simulink model "c230422_FCEV_SLMP_tbSOC_FPSD_EMS4H"  (R2022b)
settings: Solver=FixedStepAuto  StartTime=0.0  StopTime=DrvCycLen  FixedStep=1  RelTol=1e-3
values from neighbouring files (symbols this model uses):
  AccThrshd = 1    [Config_c221112.m]    (also in Config_c221127.m; Config_c221218.m; Config_c230117.m; Config_c230321.m)
  AlphaRampFactor = 8    [Config_c221112.m]    (also in Config_c221127.m; Config_c221218.m; Config_c230117.m; Config_c230321.m)
  Bat_ori_SOC2 = [0 0.001 0.002 0.003 0.004 0.005 0.006 0.007 0.008 0.009 0.01 0.011 ... (1001 elements, 1x1001)]    [FCEV_original_data.mat]
  Bat_ori_Uoc_chg_V = [2.4478 2.54923264342 2.6007 2.6383 2.66953057366 2.69636321708 2.7197 2.74042850391 2.75906114733 2.77619379074 2.792 2.80675907757 ... (1001 elements, 1x1001)]    [FCEV_original_data.mat]
  Bat_ori_Uoc_dis_V = [1.9998 2.03916768329 2.24724374236 2.39700902919 2.48767431602 2.5476 2.5882 2.6202 2.64771773167 2.6719 2.6933 2.71251566192 ... (1001 elements, 1x1001)]    [FCEV_original_data.mat]
  Bat_power_max_kW = 50    [FCEV_original_data.mat]
  Bat_power_min_kW = 0    [FCEV_original_data.mat]
  Bat_SOC_min = 0.3    [FCEV_original_data.mat]
  BattOnly = 0    [Config_c221218.m]    (also in Config_c230117.m = BattSocRightNow > BattSocLowerLimit; Config_c230321.m = double(BattSocRightNow > BattSocLowerLimit))
  BattPack_current = BattCell_current * 9    (= 20.7)    [Config_c230321.m]
  BattSocInit = 0.9    [Config_c221112.m]    (also in Config_c221127.m = 0.3; Config_c221218.m = 0.3; Config_c230117.m = 0.8; Config_c230321.m = 0.8)
  BattSocLowerLimit = 0.25    [Config_c221112.m]    (also in Config_c221127.m = 0.3; Config_c221218.m = 0.3; Config_c230117.m = 0.3; Config_c230321.m = 0.3)
  BattSocRightNow = BattSocRightNow - SocDrop    [Config_c221218.m]    (also in Config_c230117.m; Config_c230321.m)
  BattSocUpperLimit = 0.9    [Config_c221112.m]    (also in Config_c221127.m = 0.8; Config_c221218.m = 0.8; Config_c230117.m = 0.8; Config_c230321.m = 0.8)
  CFWF = 0.5    [Config_c221127.m]    (also in Config_c221218.m; Config_c230117.m; Config_c230321.m)
  DCAC_eff = 0.95    [FCEV_original_data.mat]
  DCDC_ori_eff = [0.95 0.96 0.97 0.976 0.98 0.978 0.973 0.962]    [FCEV_original_data.mat]
  DCDC_ori_power_kW = [0 10 20 30 40 50 60 70]    [FCEV_original_data.mat]
  DeAccThrshd = -1    [Config_c221112.m]    (also in Config_c221127.m; Config_c221218.m; Config_c230117.m; Config_c230321.m)
  DeltaFcPwrRcm_down = 0.5    [Config_c221127.m]    (also in Config_c221218.m; Config_c230117.m; Config_c230321.m)
  DeltaFcPwrRcm_up = 2    [Config_c221127.m]    (also in Config_c221218.m = 3; Config_c230117.m = 4; Config_c230321.m = 4)
  DrvCycRange = sum(DrvCycVps(:,2))    [Config_c221112.m]    (also in Config_c221127.m; Config_c221218.m; Config_c230117.m; Config_c230321.m)
  FC_ori_eff = [0.1 0.33 0.492 0.533 0.559 0.596 0.591 0.562 0.508]    [FCEV_original_data.mat]
  FC_ori_fuel_rate_gps = [0 0.0505050505051 0.0846883468835 0.117260787992 0.149075730471 0.279642058166 0.423011844332 0.593119810202 0.820209973753]    [FCEV_original_data.mat]
  FC_ori_power_kW = [0 2 5 7.5 10 20 30 40 50]    [FCEV_original_data.mat]
  FC_power_max_kW = 50    [FCEV_original_data.mat]
  FC_power_min_kW = 0    [FCEV_original_data.mat]
  FcPwrDropCall = 6    [Config_c221127.m]    (also in Config_c221218.m; Config_c230117.m; Config_c230321.m)
  HydpriceRmb = 30    [Config_c221127.m]    (also in Config_c221218.m; Config_c230117.m; Config_c230321.m)
  m = Time_sample    [Config_c22100601.m]    (also in Config_c22100701.m)
  MC_eff_brk_average = 0.810578512397    [FCEV_original_data.mat]
  MC_eff_dri_average = 0.810578512397    [FCEV_original_data.mat]
  MC_inertia = 0.06    [FCEV_original_data.mat]
  MC_ori_eff = [0.7 0.78 0.85 0.86 0.81 0.82 0.79 0.78 0.78 0.78 0.78 0.7 ... (231 elements, 11x21)]    [FCEV_original_data.mat]
  MC_ori_power_brk_req_kW = [0 -28.3912930389 -56.7825860779 -85.1738791168 -113.565172156 -141.956465195 -170.347758234 -198.739051273 -227.130344311 -255.52163735 -283.912930389 0 ... (121 elements, 11x11)]    [FCEV_original_data.mat]
  MC_ori_power_dri_req_kW = [0 0 0 0 0 0 0 0 0 0 0 0 ... (121 elements, 11x11)]    [FCEV_original_data.mat]
  MC_ori_spd_rpm = [0 1000 2000 3000 4000 5000 6000 7000 8000 9000 10000]    [FCEV_original_data.mat]
  MC_ori_trq_brk_max_Nm = [-271.1368 -271.1368 -271.1368 -237.5159 -178.1369 -142.4824 -118.7579 -101.8119 -89.0685 -79.172 -71.1734]    [FCEV_original_data.mat]
  MC_ori_trq_brk_Nm = [-271.136848522 -244.02316367 -216.909478817 -189.795793965 -162.682109113 -135.568424261 -108.454739409 -81.3410545565 -54.2273697044 -27.1136848522 0]    [FCEV_original_data.mat]
  MC_ori_trq_dri_max_Nm = [271.1368 271.1368 271.1368 237.5159 178.1369 142.4824 118.7579 101.8119 89.0685 79.172 71.1734]    [FCEV_original_data.mat]
  MC_ori_trq_dri_Nm = [0 27.1136848522 54.2273697044 81.3410545565 108.454739409 135.568424261 162.682109113 189.795793965 216.909478817 244.02316367 271.136848522]    [FCEV_original_data.mat]
  MC_ori_trq_Nm = [-271.136848522 -244.02316367 -216.909478817 -189.795793965 -162.682109113 -135.568424261 -108.454739409 -81.3410545565 -54.2273697044 -27.1136848522 0 27.1136848522 ... (21 elements, 1x21)]    [FCEV_original_data.mat]
  MC_power_max_kW = 75    [FCEV_original_data.mat]
  MC_spd_max_rpm = 10000    [FCEV_original_data.mat]
  MC_spd_min_rpm = 0    [FCEV_original_data.mat]
  MC_spd_scale = 1    [FCEV_original_data.mat]
  MC_trq_scale = 1    [FCEV_original_data.mat]
  nbl_std = (20/nbl_btm)^(1/0.57)    [Config_c230321.m]
  no_FcPwrSlowDrop = 1    [Config_c230321.m]
  Placeholder = 0    [Config_c221127.m]    (also in Config_c221218.m; Config_c230117.m; Config_c230321.m)
  PredLen = 5    [Config_c221112.m]    (also in Config_c221127.m; Config_c221218.m; Config_c230117.m; Config_c230321.m)
  Q_batt = 20.7*3600    (= 74520)    [Config_c22100701.m]    (also in Config_c230321.m = 18000)
  Road_u = 0.75    [FCEV_original_data.mat]
  sc_E = 0.5 * C_eff * V_eff^2    (= 512000)    [Config_c230321.m]
  SC_np = 1    [Config_c230321.m]
  SC_ns = 100    [Config_c230321.m]
  SC_rc = 1000    [Config_c230321.m]
  sc_soc_init = 0.5    [Config_c230321.m]
  SFun_ipt = [sc_discharge_limit;sc_charge_limit;sc_E;Sc_pwr_upper_lmt;BattSocLowerLimit;     BattSocUpperLimit;Q_batt;BattUoc;50;]    [Config_c230321.m]
  SLMP_LearningRate = 0.05    [Config_c221112.m]    (also in Config_c221127.m; Config_c221218.m; Config_c230117.m; Config_c230321.m)
  tDegTable = [zeros(1,3),linspace(0,0.13,47)]    [Config_c221127.m]    (also in Config_c221218.m; Config_c230117.m; Config_c230321.m)
  usd2rmb = 7.116    [Config_c22100601.m]    (also in Config_c22100701.m; Config_c221106.m = 6; Config_c221112.m = 6; Config_c221127.m = 6)
  Veh_air_density_kgpm2 = 1.2    [FCEV_original_data.mat]
  Veh_brk_front = [1 0.6 0.608 0.61 0.618 0.624 0.636 0.645 0.655]    [FCEV_original_data.mat]
  Veh_brk_z = [0.1 0.2 0.3 0.4 0.5 0.6 0.7 0.8 0.9]    [FCEV_original_data.mat]
  Veh_brk_z_max = 0.7    [FCEV_original_data.mat]
  Veh_brk_z_min = 0.1    [FCEV_original_data.mat]
  Veh_coeff_drag = 0.312    [FCEV_original_data.mat]
  Veh_coeff_roll = 0.00863    [FCEV_original_data.mat]
  Veh_final_drive_inertia = 0.1105    [FCEV_original_data.mat]
  Veh_final_drive_ratio = 3.47    [FCEV_original_data.mat]
  Veh_frontal_area_m2 = 2.06    [FCEV_original_data.mat]
  Veh_gravity_acc_ms2 = 9.81    [FCEV_original_data.mat]
  Veh_mass_cargo_kg = 113    [FCEV_original_data.mat]
  Veh_mass_curb_kg = 1157    [FCEV_original_data.mat]
  Veh_mech_eff = 0.9    [FCEV_original_data.mat]
  Veh_rotary_mass_conversion_factor = 1.05    [FCEV_original_data.mat]
  Veh_size_cg_height_m = 0.53    [FCEV_original_data.mat]
  Veh_wheel_inertia = 3.1039    [FCEV_original_data.mat]
  Veh_wheel_radius_m = 0.313    [FCEV_original_data.mat]
  Veh_wt_frac_front = 0.5    [FCEV_original_data.mat]
  VstdThrshd = 2    [Config_c221112.m]    (also in Config_c221127.m; Config_c221218.m; Config_c230117.m; Config_c230321.m)
undefined symbols (not defined in the file or in its folder): Bat_ori_temp, SC_iv, SC_nm, SC_SocTable
libraries: autolibshared x2
(part 2 of 7)

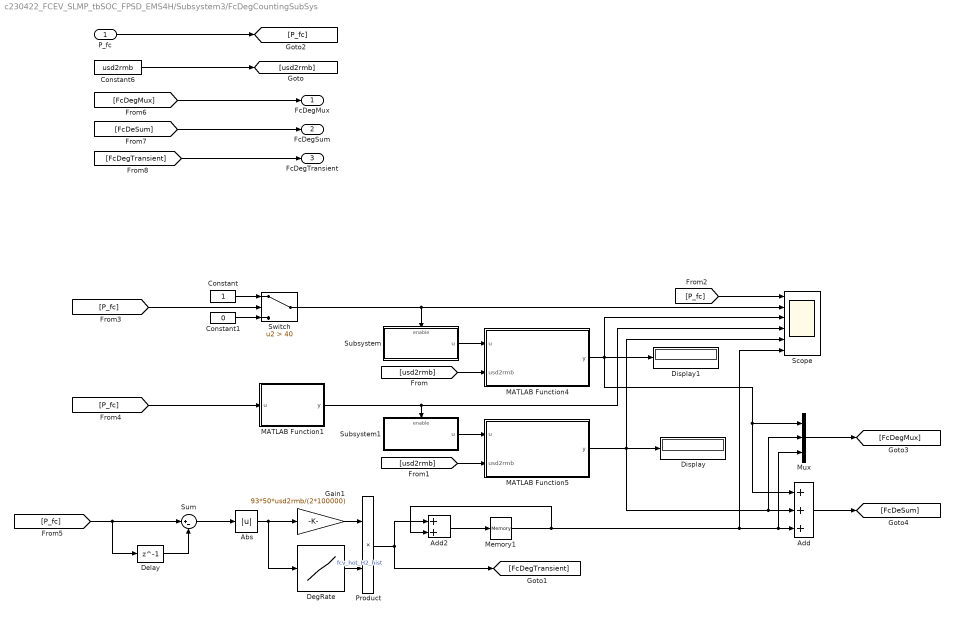
== system c230422_FCEV_SLMP_tbSOC_FPSD_EMS4H/Subsystem3/FcDegCountingSubSys ==
  P_fc : Inport
  Abs : Abs  SaturateOnIntegerOverflow=off
  Add : Sum  Inputs=+++
  Add2 : Sum
  Constant : Constant
  Constant1 : Constant  Value=0
  Constant6 : Constant  Value=usd2rmb
  DegRate : Lookup_n-D  NumberOfTableDimensions=1  BreakpointsForDimension1=1:50  Table=tDegTable  RndMeth=Simplest
  Delay : Delay  DelayLength=1
  Display : Display
  Display1 : Display
  Gain1 : Gain  Gain=93*50*usd2rmb/(2*100000)
  MATLAB Function1 : MATLAB Function  TreatAsAtomicUnit=on
  MATLAB Function4 : MATLAB Function  TreatAsAtomicUnit=on
  MATLAB Function5 : MATLAB Function  TreatAsAtomicUnit=on
  Memory1 : Memory
  Mux : Mux  Inputs=3
  Product : Product
  Scope : Scope  NumInputPorts=6
  Subsystem : Subsystem
  Subsystem1 : Subsystem
  Sum : Sum  Inputs=|+-
  Switch : Switch  Criteria=u2 > Threshold  Threshold=40  SaturateOnIntegerOverflow=off  InputSameDT=off
  FcDegMux : Outport
  FcDegSum : Outport  Port=2
  FcDegTransient : Outport  Port=3
  wires:
  MATLAB Function5/1(y) -> Scope/5, Display/1, Mux/2, Add/2
  MATLAB Function1/1(y) -> Subsystem1/Enable, Scope/4
  Subsystem/1(u) -> MATLAB Function4/1(u)
  Constant/1 -> Switch/1
  [usd2rmb] -> MATLAB Function4/2(usd2rmb)
  Constant1/1 -> Switch/3
  [usd2rmb] -> MATLAB Function5/2(usd2rmb)
  Switch/1 -> Scope/2, Subsystem/Enable
  P_fc/1 -> [P_fc]
  Subsystem1/1(u) -> MATLAB Function5/1(u)
  MATLAB Function4/1(y) -> Scope/3, Mux/1, Add/1, Display1/1
  Constant6/1 -> [usd2rmb]
  [P_fc] -> Scope/1
  Memory1/1 -> Scope/6, Mux/3, Add/3, Add2/2
  Add2/1 -> Memory1/1
  Sum/1 -> Abs/1
  Abs/1 -> DegRate/1, Gain1/1
  Delay/1 -> Sum/2
  [P_fc] -> Delay/1, Sum/1
  [P_fc] -> Switch/2
  Add/1 -> [FcDeSum]
  Mux/1 -> [FcDegMux]
  [P_fc] -> MATLAB Function1/1(u)
  [FcDegMux] -> FcDegMux/1
  [FcDeSum] -> FcDegSum/1
  [FcDegTransient] -> FcDegTransient/1
  Product/1 -> [FcDegTransient], Add2/1
  Gain1/1 -> Product/1
  DegRate/1 -> Product/2  "fcv_hot_H2_hist"

== system c230422_FCEV_SLMP_tbSOC_FPSD_EMS4H/Subsystem3/Fuel Rate Calculation1 ==
  note: Transient load response
  fc pwr : Inport
  "FC hydrogen consumption rate " : Lookup_n-D  NumberOfTableDimensions=1  BreakpointsForDimension1=FC_ori_power_kW  Table=FC_ori_fuel_rate_gps  RndMeth=Simplest
  fcv_H2_rate (g/s)1 : Outport
  wires:
  fc pwr/1 -> "FC hydrogen consumption rate "/1
  "FC hydrogen consumption rate "/1 -> fcv_H2_rate (g/s)1/1  "fcv_hot_H2_hist"

== system c230422_FCEV_SLMP_tbSOC_FPSD_EMS4H/Subsystem3/Fuel cell efficiency calculation ==
  note: Carryover
  note: Transient load response
  fc power : Inport
  "FC efficiency " : Lookup_n-D  NumberOfTableDimensions=1  BreakpointsForDimension1=FC_ori_power_kW  Table=FC_ori_eff  RndMeth=Simplest
  "fc_eff " : Outport
  wires:
  "FC efficiency "/1 -> "fc_eff "/1
  fc power/1 -> "FC efficiency "/1

== system c230422_FCEV_SLMP_tbSOC_FPSD_EMS4H/Subsystem3/Power Calculation ==
  note: Transient load response
  fc on : Inport
  Power command (kW) : Inport  Port=2
  "   " : Constant  Value=0
  Switch2 : Switch  Threshold=0.5
  Power output (kW) : Outport
  wires:
  "   "/1 -> Switch2/3
  Power command (kW)/1 -> Switch2/1
  fc on/1 -> Switch2/2
  Switch2/1 -> Power output (kW)/1

== system c230422_FCEV_SLMP_tbSOC_FPSD_EMS4H/Subsystem4/VehModel_Pred+1 ==
  note: CarryOver
  Pred_v1 : Inport
  Enable : EnablePort
  Gain : Gain  Gain=3.6
  Power bus : Subsystem
  主减及变速器模型 : Subsystem
  整车动力学模型 : Subsystem
  车轮模型 : Subsystem
  驱动电机模型 : Subsystem
  PredPwr_1 : Outport
  wires:
  主减及变速器模型/1(drive torque (Nm) speed (rad/s) brike torque (Nm) req'd at input side of final drive) -> 驱动电机模型/1(drive torque (Nm) speed (rad/s) brake torque (Nm) req'd at motor)
  驱动电机模型/1(drive power (kW) brake power (kW) req'd motor input power (电功率)) -> Power bus/1(drive power (kW) brake power (kW) req at power bus)
  整车动力学模型/1(需求驱动力N 目标车速m/s 需求制动力N) -> 车轮模型/1("tractive force, brake force and speed req'd of tire/road interface 需求驱动力N 目标车速m/s 需求制动力N")
  车轮模型/1(drive torque (Nm) speed (rad/s) brake torque (Nm) req'd from drivetrain into axle) -> 主减及变速器模型/1(drive torque (Nm) speed (rad/s) brake torque (Nm) req'd at output side of final drive)
  Pred_v1/1 -> Gain/1
  Power bus/1(drive power (kW)/brake power (kW) req from power sources) -> PredPwr_1/1
  Gain/1 -> 整车动力学模型/1(需求车速 km/h)

== system c230422_FCEV_SLMP_tbSOC_FPSD_EMS4H/Subsystem4/VehModel_Pred+2 ==
  note: CarryOver
  Pred_v2 : Inport
  Pred_v1 : Inport  Port=2
  Enable : EnablePort
  Gain : Gain  Gain=3.6
  Gain1 : Gain  Gain=3.6
  Power bus : Subsystem
  主减及变速器模型 : Subsystem
  整车动力学模型 : Subsystem
  车轮模型 : Subsystem
  驱动电机模型 : Subsystem
  PredPwr_2 : Outport
  wires:
  主减及变速器模型/1(drive torque (Nm) speed (rad/s) brike torque (Nm) req'd at input side of final drive) -> 驱动电机模型/1(drive torque (Nm) speed (rad/s) brake torque (Nm) req'd at motor)
  驱动电机模型/1(drive power (kW) brake power (kW) req'd motor input power (电功率)) -> Power bus/1(drive power (kW) brake power (kW) req at power bus)
  整车动力学模型/1(需求驱动力N 目标车速m/s 需求制动力N) -> 车轮模型/1("tractive force, brake force and speed req'd of tire/road interface 需求驱动力N 目标车速m/s 需求制动力N")
  车轮模型/1(drive torque (Nm) speed (rad/s) brake torque (Nm) req'd from drivetrain into axle) -> 主减及变速器模型/1(drive torque (Nm) speed (rad/s) brake torque (Nm) req'd at output side of final drive)
  Pred_v2/1 -> Gain/1
  Power bus/1(drive power (kW)/brake power (kW) req from power sources) -> PredPwr_2/1
  Gain/1 -> 整车动力学模型/1(需求车速 km/h)
  Pred_v1/1 -> Gain1/1
  Gain1/1 -> 整车动力学模型/2(Temp)

== system c230422_FCEV_SLMP_tbSOC_FPSD_EMS4H/Subsystem4/VehModel_Pred+3 ==
  note: CarryOver
  Pred_v3 : Inport
  Pred_v2 : Inport  Port=2
  Enable : EnablePort
  Gain : Gain  Gain=3.6
  Gain1 : Gain  Gain=3.6
  Power bus : Subsystem
  主减及变速器模型 : Subsystem
  整车动力学模型 : Subsystem
  车轮模型 : Subsystem
  驱动电机模型 : Subsystem
  PredPwr_3 : Outport
  wires:
  主减及变速器模型/1(drive torque (Nm) speed (rad/s) brike torque (Nm) req'd at input side of final drive) -> 驱动电机模型/1(drive torque (Nm) speed (rad/s) brake torque (Nm) req'd at motor)
  驱动电机模型/1(drive power (kW) brake power (kW) req'd motor input power (电功率)) -> Power bus/1(drive power (kW) brake power (kW) req at power bus)
  整车动力学模型/1(需求驱动力N 目标车速m/s 需求制动力N) -> 车轮模型/1("tractive force, brake force and speed req'd of tire/road interface 需求驱动力N 目标车速m/s 需求制动力N")
  车轮模型/1(drive torque (Nm) speed (rad/s) brake torque (Nm) req'd from drivetrain into axle) -> 主减及变速器模型/1(drive torque (Nm) speed (rad/s) brake torque (Nm) req'd at output side of final drive)
  Pred_v3/1 -> Gain/1
  Power bus/1(drive power (kW)/brake power (kW) req from power sources) -> PredPwr_3/1
  Gain/1 -> 整车动力学模型/1(需求车速 km/h)
  Pred_v2/1 -> Gain1/1
  Gain1/1 -> 整车动力学模型/2(需求车速 km/h1)

== system c230422_FCEV_SLMP_tbSOC_FPSD_EMS4H/Subsystem4/VehModel_Pred+4 ==
  note: CarryOver
  Pred_v4 : Inport
  Pred_v3 : Inport  Port=2
  Enable : EnablePort
  Gain : Gain  Gain=3.6
  Gain1 : Gain  Gain=3.6
  Power bus : Subsystem
  主减及变速器模型 : Subsystem
  整车动力学模型 : Subsystem
  车轮模型 : Subsystem
  驱动电机模型 : Subsystem
  PredPwr_4 : Outport
  wires:
  主减及变速器模型/1(drive torque (Nm) speed (rad/s) brike torque (Nm) req'd at input side of final drive) -> 驱动电机模型/1(drive torque (Nm) speed (rad/s) brake torque (Nm) req'd at motor)
  驱动电机模型/1(drive power (kW) brake power (kW) req'd motor input power (电功率)) -> Power bus/1(drive power (kW) brake power (kW) req at power bus)
  整车动力学模型/1(需求驱动力N 目标车速m/s 需求制动力N) -> 车轮模型/1("tractive force, brake force and speed req'd of tire/road interface 需求驱动力N 目标车速m/s 需求制动力N")
  车轮模型/1(drive torque (Nm) speed (rad/s) brake torque (Nm) req'd from drivetrain into axle) -> 主减及变速器模型/1(drive torque (Nm) speed (rad/s) brake torque (Nm) req'd at output side of final drive)
  Pred_v4/1 -> Gain/1
  Power bus/1(drive power (kW)/brake power (kW) req from power sources) -> PredPwr_4/1
  Gain/1 -> 整车动力学模型/1(需求车速 km/h)
  Pred_v3/1 -> Gain1/1
  Gain1/1 -> 整车动力学模型/2(需求车速 km/h1)

== system c230422_FCEV_SLMP_tbSOC_FPSD_EMS4H/Subsystem4/VehModel_Pred+5 ==
  note: CarryOver
  Pred_v5 : Inport
  Pred_v4 : Inport  Port=2
  Enable : EnablePort
  Gain : Gain  Gain=3.6
  Gain1 : Gain  Gain=3.6
  Power bus : Subsystem
  主减及变速器模型 : Subsystem
  整车动力学模型 : Subsystem
  车轮模型 : Subsystem
  驱动电机模型 : Subsystem
  PredPwr_5 : Outport
  wires:
  主减及变速器模型/1(drive torque (Nm) speed (rad/s) brike torque (Nm) req'd at input side of final drive) -> 驱动电机模型/1(drive torque (Nm) speed (rad/s) brake torque (Nm) req'd at motor)
  驱动电机模型/1(drive power (kW) brake power (kW) req'd motor input power (电功率)) -> Power bus/1(drive power (kW) brake power (kW) req at power bus)
  整车动力学模型/1(需求驱动力N 目标车速m/s 需求制动力N) -> 车轮模型/1("tractive force, brake force and speed req'd of tire/road interface 需求驱动力N 目标车速m/s 需求制动力N")
  车轮模型/1(drive torque (Nm) speed (rad/s) brake torque (Nm) req'd from drivetrain into axle) -> 主减及变速器模型/1(drive torque (Nm) speed (rad/s) brake torque (Nm) req'd at output side of final drive)
  Pred_v5/1 -> Gain/1
  Power bus/1(drive power (kW)/brake power (kW) req from power sources) -> PredPwr_5/1
  Gain/1 -> 整车动力学模型/1(需求车速 km/h)
  Pred_v4/1 -> Gain1/1
  Gain1/1 -> 整车动力学模型/2(需求车速 km/h1)

== system c230422_FCEV_SLMP_tbSOC_FPSD_EMS4H/Subsystem4/VehModel_Pred+6 ==
  note: CarryOver
  Pred_v6 : Inport
  Pred_v5 : Inport  Port=2
  Enable : EnablePort
  Gain : Gain  Gain=3.6
  Gain1 : Gain  Gain=3.6
  Power bus : Subsystem
  主减及变速器模型 : Subsystem
  整车动力学模型 : Subsystem
  车轮模型 : Subsystem
  驱动电机模型 : Subsystem
  PredPwr_6 : Outport
  wires:
  Gain/1 -> 整车动力学模型/1(需求车速 km/h)
  Power bus/1(drive power (kW)/brake power (kW) req from power sources) -> PredPwr_6/1
  Pred_v6/1 -> Gain/1
  车轮模型/1(drive torque (Nm) speed (rad/s) brake torque (Nm) req'd from drivetrain into axle) -> 主减及变速器模型/1(drive torque (Nm) speed (rad/s) brake torque (Nm) req'd at output side of final drive)
  整车动力学模型/1(需求驱动力N 目标车速m/s 需求制动力N) -> 车轮模型/1("tractive force, brake force and speed req'd of tire/road interface 需求驱动力N 目标车速m/s 需求制动力N")
  驱动电机模型/1(drive power (kW) brake power (kW) req'd motor input power (电功率)) -> Power bus/1(drive power (kW) brake power (kW) req at power bus)
  主减及变速器模型/1(drive torque (Nm) speed (rad/s) brike torque (Nm) req'd at input side of final drive) -> 驱动电机模型/1(drive torque (Nm) speed (rad/s) brake torque (Nm) req'd at motor)
  Pred_v5/1 -> Gain1/1
  Gain1/1 -> 整车动力学模型/2(需求车速 km/h1)

== system c230422_FCEV_SLMP_tbSOC_FPSD_EMS4H/Subsystem4/VehModel_Pred+7 ==
  note: CarryOver
  Pred_v7 : Inport
  Pred_v6 : Inport  Port=2
  Enable : EnablePort
  Gain : Gain  Gain=3.6
  Gain1 : Gain  Gain=3.6
  Power bus : Subsystem
  主减及变速器模型 : Subsystem
  整车动力学模型 : Subsystem
  车轮模型 : Subsystem
  驱动电机模型 : Subsystem
  PredPwr_7 : Outport
  wires:
  Gain/1 -> 整车动力学模型/1(需求车速 km/h)
  Power bus/1(drive power (kW)/brake power (kW) req from power sources) -> PredPwr_7/1
  Pred_v7/1 -> Gain/1
  车轮模型/1(drive torque (Nm) speed (rad/s) brake torque (Nm) req'd from drivetrain into axle) -> 主减及变速器模型/1(drive torque (Nm) speed (rad/s) brake torque (Nm) req'd at output side of final drive)
  整车动力学模型/1(需求驱动力N 目标车速m/s 需求制动力N) -> 车轮模型/1("tractive force, brake force and speed req'd of tire/road interface 需求驱动力N 目标车速m/s 需求制动力N")
  驱动电机模型/1(drive power (kW) brake power (kW) req'd motor input power (电功率)) -> Power bus/1(drive power (kW) brake power (kW) req at power bus)
  主减及变速器模型/1(drive torque (Nm) speed (rad/s) brike torque (Nm) req'd at input side of final drive) -> 驱动电机模型/1(drive torque (Nm) speed (rad/s) brake torque (Nm) req'd at motor)
  Pred_v6/1 -> Gain1/1
  Gain1/1 -> 整车动力学模型/2(需求车速 km/h1)

== system c230422_FCEV_SLMP_tbSOC_FPSD_EMS4H/Subsystem4/VehModel_Pred+8 ==
  note: CarryOver
  Pred_v8 : Inport
  Pred_v7 : Inport  Port=2
  Enable : EnablePort
  Gain : Gain  Gain=3.6
  Gain1 : Gain  Gain=3.6
  Power bus : Subsystem
  主减及变速器模型 : Subsystem
  整车动力学模型 : Subsystem
  车轮模型 : Subsystem
  驱动电机模型 : Subsystem
  PredPwr_8 : Outport
  wires:
  Gain/1 -> 整车动力学模型/1(需求车速 km/h)
  Power bus/1(drive power (kW)/brake power (kW) req from power sources) -> PredPwr_8/1
  Pred_v8/1 -> Gain/1
  车轮模型/1(drive torque (Nm) speed (rad/s) brake torque (Nm) req'd from drivetrain into axle) -> 主减及变速器模型/1(drive torque (Nm) speed (rad/s) brake torque (Nm) req'd at output side of final drive)
  整车动力学模型/1(需求驱动力N 目标车速m/s 需求制动力N) -> 车轮模型/1("tractive force, brake force and speed req'd of tire/road interface 需求驱动力N 目标车速m/s 需求制动力N")
  驱动电机模型/1(drive power (kW) brake power (kW) req'd motor input power (电功率)) -> Power bus/1(drive power (kW) brake power (kW) req at power bus)
  主减及变速器模型/1(drive torque (Nm) speed (rad/s) brike torque (Nm) req'd at input side of final drive) -> 驱动电机模型/1(drive torque (Nm) speed (rad/s) brake torque (Nm) req'd at motor)
  Pred_v7/1 -> Gain1/1
  Gain1/1 -> 整车动力学模型/2(需求车速 km/h1)

== system c230422_FCEV_SLMP_tbSOC_FPSD_EMS4H/Subsystem4/VehModel_Pred+9 ==
  note: CarryOver
  Pred_v9 : Inport
  Pred_v8 : Inport  Port=2
  Enable : EnablePort
  Gain : Gain  Gain=3.6
  Gain1 : Gain  Gain=3.6
  Power bus : Subsystem
  主减及变速器模型 : Subsystem
  整车动力学模型 : Subsystem
  车轮模型 : Subsystem
  驱动电机模型 : Subsystem
  PredPwr_9 : Outport
  wires:
  Gain/1 -> 整车动力学模型/1(需求车速 km/h)
  Power bus/1(drive power (kW)/brake power (kW) req from power sources) -> PredPwr_9/1
  Pred_v9/1 -> Gain/1
  车轮模型/1(drive torque (Nm) speed (rad/s) brake torque (Nm) req'd from drivetrain into axle) -> 主减及变速器模型/1(drive torque (Nm) speed (rad/s) brake torque (Nm) req'd at output side of final drive)
  整车动力学模型/1(需求驱动力N 目标车速m/s 需求制动力N) -> 车轮模型/1("tractive force, brake force and speed req'd of tire/road interface 需求驱动力N 目标车速m/s 需求制动力N")
  驱动电机模型/1(drive power (kW) brake power (kW) req'd motor input power (电功率)) -> Power bus/1(drive power (kW) brake power (kW) req at power bus)
  主减及变速器模型/1(drive torque (Nm) speed (rad/s) brike torque (Nm) req'd at input side of final drive) -> 驱动电机模型/1(drive torque (Nm) speed (rad/s) brake torque (Nm) req'd at motor)
  Pred_v8/1 -> Gain1/1
  Gain1/1 -> 整车动力学模型/2(需求车速 km/h1)

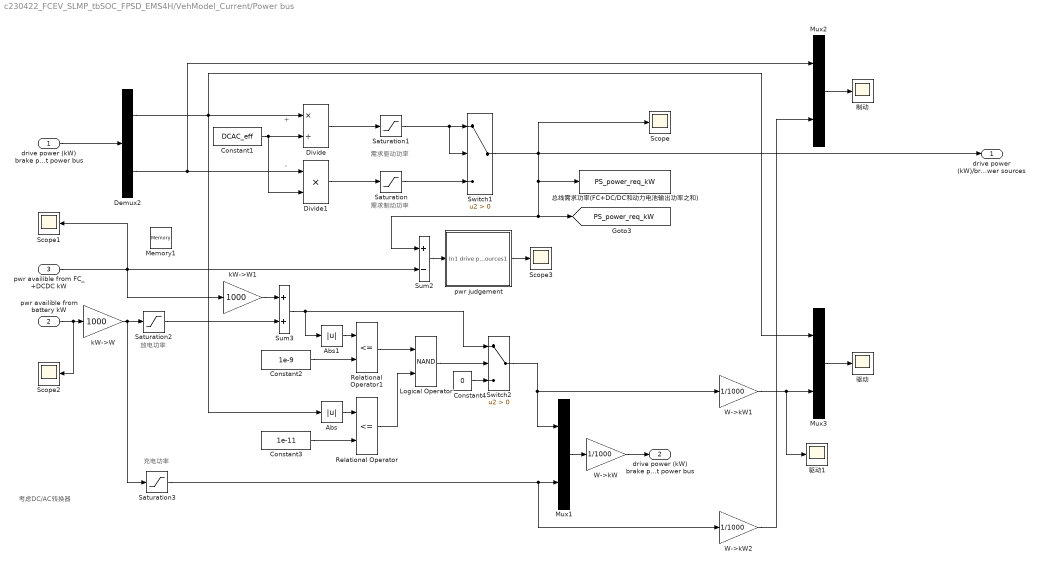
== system c230422_FCEV_SLMP_tbSOC_FPSD_EMS4H/VehModel_Current/Power bus ==
  note: 充电功率
  note: 放电功率
  note: 考虑DC/AC转换器
  note: -
  note: +
  note: 需求制动功率
  note: 需求驱动功率
  drive power (kW) brake power (kW) req at power bus : Inport
  pwr availible from battery kW : Inport  Port=2
  pwr availible from FC_+DCDC kW : Inport  Port=3
  Abs : Abs  SaturateOnIntegerOverflow=off
  Abs1 : Abs  SaturateOnIntegerOverflow=off
  Constant1 : Constant  Value=DCAC_eff
  Constant2 : Constant  Value=1e-9
  Constant3 : Constant  Value=1e-11
  Constant4 : Constant  Value=0
  Demux2 : Demux  Outputs=2
  Divide : Product  Inputs=*/
  Divide1 : Product  Inputs=**
  Logical Operator : Logic  Operator=NAND  AllPortsSameDT=off  OutDataTypeStr=boolean
  Memory1 : Memory  InheritSampleTime=on
  Mux1 : Mux  Inputs=2
  Mux2 : Mux  Inputs=2
  Mux3 : Mux  Inputs=2
  Relational Operator : RelationalOperator  Operator=<=  OutDataTypeStr=boolean  InputSameDT=off
  Relational Operator1 : RelationalOperator  Operator=<=  OutDataTypeStr=boolean  InputSameDT=off
  Saturation : Saturate  UpperLimit=0  LowerLimit=-inf
  Saturation1 : Saturate  UpperLimit=inf  LowerLimit=0
  Saturation2 : Saturate  UpperLimit=inf  LowerLimit=0
  Saturation3 : Saturate  UpperLimit=0  LowerLimit=-inf
  Scope{,1..3} (4 alike) : Scope
  Sum2 : Sum  Inputs=+-
  Sum3 : Sum
  Switch1 : Switch  Criteria=u2 > Threshold  SaturateOnIntegerOverflow=off  InputSameDT=off
  Switch2 : Switch  Criteria=u2 > Threshold  SaturateOnIntegerOverflow=off  InputSameDT=off
  W->kW : Gain  Gain=1/1000
  W->kW1 : Gain  Gain=1/1000
  W->kW2 : Gain  Gain=1/1000
  kW->W : Gain  Gain=1000
  kW->W1 : Gain  Gain=1000
  pwr judgement : Subsystem
  制动 : Scope
  总线需求功率(FC+DC/DC和动力电池输出功率之和) : ToWorkspace  VariableName=PS_power_req_kW  SampleTime=-1
  驱动 : Scope
  驱动1 : Scope
  drive power (kW)/brake power (kW) req from power sources : Outport
  drive power (kW) brake power (kW) availableat power bus : Outport  Port=2
  tag scope: PS_power_req_kW=global
  wires:
  Abs1/1 -> Relational Operator1/1
  Constant2/1 -> Relational Operator1/2
  Constant1/1 -> Divide1/2, Divide/2
  Divide/1 -> Saturation1/1
  Divide1/1 -> Saturation/1
  drive power (kW) brake power (kW) req at power bus/1 -> Demux2/1
  Demux2/2 -> Mux2/1, Divide1/1
  Saturation1/1 -> Switch1/2, Switch1/1
  Switch1/1 -> drive power (kW)/brake power (kW) req from power sources/1, 总线需求功率(FC+DC/DC和动力电池输出功率之和)/1, Sum2/1, [PS_power_req_kW], Scope/1
  W->kW/1 -> drive power (kW) brake power (kW) availableat power bus/1
  Saturation/1 -> Switch1/3
  Mux2/1 -> 制动/1
  Mux3/1 -> 驱动/1
  W->kW1/1 -> 驱动1/1, Mux3/2
  W->kW2/1 -> Mux2/2
  Sum2/1 -> pwr judgement/1(In1)
  Saturation2/1 -> Sum3/2
  pwr availible from FC_+DCDC kW/1 -> kW->W1/1, Scope1/1, Sum2/2
  Sum3/1 -> Switch2/1, Abs1/1
  Relational Operator1/1 -> Logical Operator/1
  Abs/1 -> Relational Operator/1
  Constant3/1 -> Relational Operator/2
  Demux2/1 -> Mux3/1, Abs/1, Divide/1
  Relational Operator/1 -> Logical Operator/2
  Constant4/1 -> Switch2/3
  Logical Operator/1 -> Switch2/2
  Saturation3/1 -> W->kW2/1, Mux1/2
  Switch2/1 -> W->kW1/1, Mux1/1
  pwr availible from battery kW/1 -> Scope2/1, kW->W/1
  kW->W/1 -> Saturation3/1, Saturation2/1
  kW->W1/1 -> Sum3/1
  Mux1/1 -> W->kW/1
  pwr judgement/1(drive power (kW)/brake power (kW) req from power sources1) -> Scope3/1

== system c230422_FCEV_SLMP_tbSOC_FPSD_EMS4H/VehModel_Current/主减及变速器模型 ==
  drive torque (Nm) speed (rad/s) brake torque (Nm) req'd at output side of final drive : Inport
  drive torque (Nm) brake torque (Nm) speed avail (rad/s) at input side of final drive : Inport  Port=2
  " Effect of inertia (Nm)1" : Subsystem
  Demux1 : Demux  Outputs=3
  Demux4 : Demux  Outputs=3
  Effect of inertia (Nm) : Subsystem
  Gain1 : Gain  Gain=1/Veh_final_drive_ratio
  Gain2 : Gain  Gain=1/Veh_final_drive_ratio
  Gain3 : Gain  Gain=Veh_final_drive_ratio  SaturateOnIntegerOverflow=on  OutDataTypeStr=Inherit: Same as input  ParamDataTypeStr=Inherit: Same as input
  Gain4 : Gain  Gain=1/Veh_final_drive_ratio  SaturateOnIntegerOverflow=on  OutDataTypeStr=Inherit: Same as input  ParamDataTypeStr=Inherit: Same as input
  Gain5 : Gain  Gain=Veh_final_drive_ratio  SaturateOnIntegerOverflow=on  OutDataTypeStr=Inherit: Same as input  ParamDataTypeStr=Inherit: Same as input
  Gain8 : Gain  Gain=Veh_final_drive_ratio  SaturateOnIntegerOverflow=on  OutDataTypeStr=Inherit: Same as input  ParamDataTypeStr=Inherit: Same as input
  Mux1 : Mux  Inputs=3
  Mux4 : Mux  Inputs=3
  Saturation : Saturate  UpperLimit=inf  LowerLimit=0
  Saturation1 : Saturate  UpperLimit=0  LowerLimit=-inf
  Saturation2 : Saturate  UpperLimit=inf  LowerLimit=0
  Scope : Scope
  Sum : Sum  Inputs=+++  InputSameDT=on  SaturateOnIntegerOverflow=on  OutDataTypeStr=Inherit: Same as first input
  Sum2 : Sum  Inputs=--+  InputSameDT=on  SaturateOnIntegerOverflow=on  OutDataTypeStr=Inherit: Same as first input
  Sum3 : Sum  Inputs=+++  InputSameDT=on  SaturateOnIntegerOverflow=on  OutDataTypeStr=Inherit: Same as first input
  Sum4 : Sum  Inputs=--+  InputSameDT=on  SaturateOnIntegerOverflow=on  OutDataTypeStr=Inherit: Same as first input
  loss (Nm) : Subsystem
  loss (Nm)1 : Subsystem
  主减速器需求制动转矩 : Scope
  主减速器需求转速 : Scope
  主减速器需求驱动转矩 : Scope
  drive torque (Nm) speed (rad/s) brike torque (Nm) req'd at input side of final drive : Outport  InitialOutput=0
  drive torque (Nm) brake torque (Nm) speed avail (rad/s) at output side of final drive : Outport  Port=2  InitialOutput=0
  wires:
  Demux4/2 -> Effect of inertia (Nm)/1(fd input speed (rad/s)), " Effect of inertia (Nm)1"/1(In1), Gain3/1
  Demux4/1 -> loss (Nm)/1("drive torque (Nm) "), Gain1/1
  Mux4/1 -> drive torque (Nm) speed (rad/s) brike torque (Nm) req'd at input side of final drive/1
  drive torque (Nm) speed (rad/s) brake torque (Nm) req'd at output side of final drive/1 -> Demux4/1
  Mux1/1 -> Scope/1, drive torque (Nm) brake torque (Nm) speed avail (rad/s) at output side of final drive/1
  drive torque (Nm) brake torque (Nm) speed avail (rad/s) at input side of final drive/1 -> Demux1/1
  Effect of inertia (Nm)/1(drag torque (Nm)) -> Sum2/2, Sum/2
  loss (Nm)/1(drag torque (Nm)) -> Sum2/1, Sum/1
  Gain1/1 -> Sum/3
  Sum/1 -> 主减速器需求驱动转矩/1, Mux4/1
  Gain3/1 -> 主减速器需求转速/1, Mux4/2
  " Effect of inertia (Nm)1"/1(Out1) -> Sum4/1, Sum3/2
  loss (Nm)1/1(drag torque (Nm)) -> Sum4/2, Sum3/3
  Demux4/3 -> Gain2/1, loss (Nm)1/1("drive torque (Nm) ")
  Gain2/1 -> Sum3/1
  Demux1/1 -> Sum2/3
  Demux1/2 -> Sum4/3
  Sum2/1 -> Gain8/1
  Gain8/1 -> Saturation/1
  Saturation/1 -> Mux1/1
  Sum4/1 -> Gain5/1
  Saturation1/1 -> Mux1/2
  Gain5/1 -> Saturation1/1
  Gain4/1 -> Saturation2/1
  Demux1/3 -> Gain4/1
  Saturation2/1 -> Mux1/3
  Sum3/1 -> 主减速器需求制动转矩/1, Mux4/3

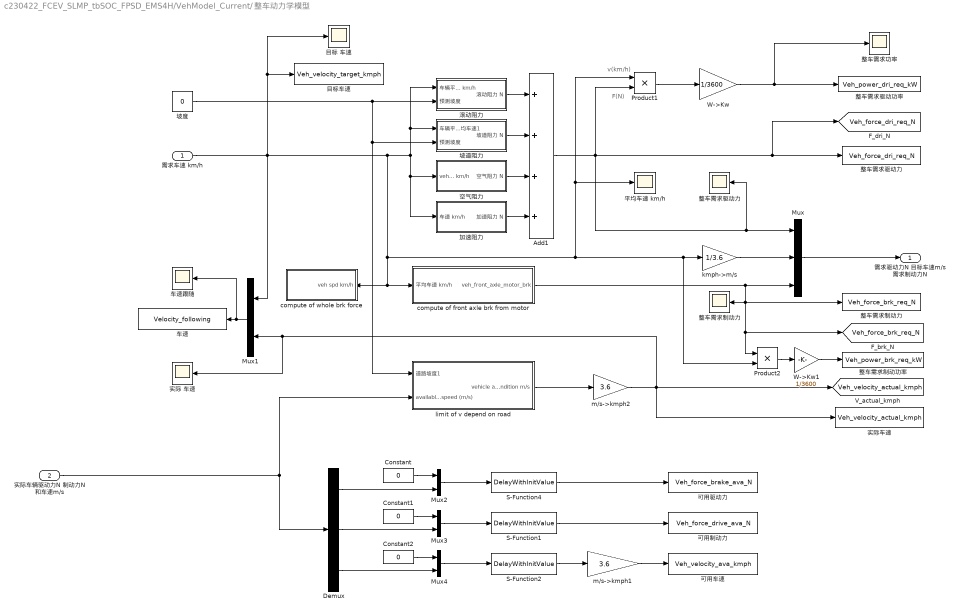
== system c230422_FCEV_SLMP_tbSOC_FPSD_EMS4H/VehModel_Current/整车动力学模型 ==
  note: v(km/h)
  note: F(N)
  需求车速 km/h : Inport
  实际车辆驱动力N 制动力N 和车速m/s : Inport  Port=2
  "  整车需求制动力" : ToWorkspace  VariableName=Veh_force_brk_req_N  SaveFormat=Timeseries  SampleTime=-1
  "  整车需求制动功率" : ToWorkspace  VariableName=Veh_power_brk_req_kW  SampleTime=-1
  "  整车需求驱动力" : ToWorkspace  VariableName=Veh_force_dri_req_N  SaveFormat=Timeseries  SampleTime=-1
  "  整车需求驱动功率" : ToWorkspace  VariableName=Veh_power_dri_req_kW  SampleTime=-1
  "  目标车速" : ToWorkspace  VariableName=Veh_velocity_target_kmph  SaveFormat=Timeseries  SampleTime=-1
  "  车速" : ToWorkspace  VariableName=Velocity_following  SaveFormat=Timeseries  SampleTime=-1
  Add1 : Sum  Inputs=++++
  Constant : Constant  Value=0
  Constant1 : Constant  Value=0
  Constant2 : Constant  Value=0
  Demux : Demux  Outputs=3
  Mux : Mux  Inputs=3
  Mux{1..4} (4 alike) : Mux  Inputs=2
  Product1 : Product  RndMeth=Zero
  Product2 : Product  RndMeth=Zero
  S-Function1 : S-Function  FunctionName=DelayWithInitValue  SFunctionDeploymentMode=off  EnableBusSupport=off
  S-Function2 : S-Function  FunctionName=DelayWithInitValue  SFunctionDeploymentMode=off  EnableBusSupport=off
  S-Function4 : S-Function  FunctionName=DelayWithInitValue  SFunctionDeploymentMode=off  EnableBusSupport=off
  W->Kw : Gain  Gain=1/3600
  W->Kw1 : Gain  Gain=1/3600
  compute of front axle brk from motor : Subsystem
  compute of whole brk force : Subsystem
  kmph->m/s : Gain  Gain=1/3.6
  limit of v depend on road : Subsystem
  m/s->kmph1 : Gain  Gain=3.6
  m/s->kmph2 : Gain  Gain=3.6
  加速阻力 : Subsystem
  可用制动力 : ToWorkspace  VariableName=Veh_force_drive_ava_N  SaveFormat=Timeseries  SampleTime=-1
  可用车速 : ToWorkspace  VariableName=Veh_velocity_ava_kmph  SaveFormat=Timeseries  SampleTime=-1
  可用驱动力 : ToWorkspace  VariableName=Veh_force_brake_ava_N  SaveFormat=Timeseries  SampleTime=-1
  坡度 : Constant  Value=0
  坡道阻力 : Subsystem
  实际 车速 : Scope
  实际车速 : ToWorkspace  VariableName=Veh_velocity_actual_kmph  SaveFormat=Timeseries  SampleTime=-1
  平均车速 km/h : Scope
  整车需求制动力 : Scope
  整车需求功率 : Scope
  整车需求驱动力 : Scope
  滚动阻力 : Subsystem
  目标 车速 : Scope
  空气阻力 : Subsystem
  车速跟随 : Scope
  需求驱动力N 目标车速m/s 需求制动力N : Outport
  tag scope: Veh_force_brk_req_N=global, Veh_force_dri_req_N=global, Veh_velocity_actual_kmph=global
  wires:
  实际车辆驱动力N 制动力N 和车速m/s/1 -> limit of v depend on road/2(available drive force (N) brake force (N) and linear speed (m/s)), Demux/1
  滚动阻力/1(滚动阻力 N) -> Add1/1
  坡道阻力/1(坡道阻力 N) -> Add1/2
  空气阻力/1(空气阻力 N) -> Add1/3
  加速阻力/1(加速阻力 N) -> Add1/4
  Add1/1 -> 整车需求驱动力/1, Mux/1, [Veh_force_dri_req_N], "  整车需求驱动力"/1, Product1/2
  Mux/1 -> 需求驱动力N 目标车速m/s 需求制动力N/1
  Product1/1 -> W->Kw/1
  Demux/1 -> Mux2/2
  坡度/1 -> limit of v depend on road/1(道路坡度1), 坡道阻力/2(预测坡度), 滚动阻力/2(预测坡度)
  W->Kw/1 -> "  整车需求驱动功率"/1, 整车需求功率/1
  kmph->m/s/1 -> Mux/2
  limit of v depend on road/1(vehicle achievable consider of the road condition m/s) -> m/s->kmph2/1
  m/s->kmph2/1 -> 实际车速/1, Mux1/2, 实际 车速/1, [Veh_velocity_actual_kmph]
  需求车速 km/h/1 -> 目标 车速/1, "  目标车速"/1, compute of front axle brk from motor/1(平均车速 km/h), compute of whole brk force/1(veh spd km/h), Product2/2, kmph->m/s/1, 平均车速 km/h/1, Product1/1, 加速阻力/1(车速 km/h), 空气阻力/1(veh_spd km/h), 滚动阻力/1(车辆平均车速 km/h), 坡道阻力/1(车辆平均车速1), Mux1/1
  m/s->kmph1/1 -> 可用车速/1
  compute of front axle brk from motor/1(veh_front_axle_motor_brk) -> Mux/3, 整车需求制动力/1, "  整车需求制动力"/1, [Veh_force_brk_req_N], Product2/1
  Product2/1 -> W->Kw1/1
  W->Kw1/1 -> "  整车需求制动功率"/1
  Demux/3 -> Mux4/2
  Demux/2 -> Mux3/2
  Mux1/1 -> "  车速"/1, 车速跟随/1
  Constant/1 -> Mux2/1
  Mux2/1 -> S-Function4/1
  S-Function4/1 -> 可用驱动力/1
  Mux3/1 -> S-Function1/1
  Constant1/1 -> Mux3/1
  Constant2/1 -> Mux4/1
  Mux4/1 -> S-Function2/1
  S-Function1/1 -> 可用制动力/1
  S-Function2/1 -> m/s->kmph1/1

== system c230422_FCEV_SLMP_tbSOC_FPSD_EMS4H/VehModel_Current/车轮模型 ==
  "tractive force, brake force and speed req'd of tire/road interface 需求驱动力N 目标车速m/s 需求制动力N" : Inport
  "drive torque (Nm) brake torque (Nm) speed (rad/s) available from drivetrain into axle " : Inport  Port=2
  - : Gain  Gain=Veh_wheel_radius_m
  Add : Sum
  Add1 : Sum
  Add2 : Sum  Inputs=-+
  Add3 : Sum  Inputs=-+
  Constant : Constant  Value=0
  Demux : Demux  Outputs=3
  Demux1 : Demux  Outputs=3
  Gain1 : Gain  Gain=Veh_wheel_radius_m
  Gain2 : Gain  Gain=1/Veh_wheel_radius_m
  Gain3 : Gain  Gain=1/Veh_wheel_radius_m
  Gain4 : Gain  Gain=Veh_wheel_radius_m
  Interia torque : Subsystem
  Interia torque1 : Subsystem
  Mux : Mux  Inputs=3
  Mux3 : Mux  Inputs=3
  Regenerative energy compute : Subsystem
  Saturation : Saturate  UpperLimit=inf  LowerLimit=0
  Saturation1 : Saturate  UpperLimit=0  LowerLimit=-inf
  Scope : Scope
  Switch1 : Switch  Criteria=u2 > Threshold  Threshold=15  SaturateOnIntegerOverflow=off  InputSameDT=off
  Tire slip model : Subsystem
  Tire slip model1 : Subsystem
  axle input speed (rad/s) : Gain  Gain=1/Veh_wheel_radius_m
  drive torque (Nm) speed (rad/s) brake torque (Nm) req'd from drivetrain into axle : Outport  InitialOutput=0
  tractive force (N) brake force (N) linear speed achievable (m/s) : Outport  Port=2  InitialOutput=0
  wires:
  Demux/1 -> Gain1/1
  "tractive force, brake force and speed req'd of tire/road interface 需求驱动力N 目标车速m/s 需求制动力N"/1 -> Demux/1
  "drive torque (Nm) brake torque (Nm) speed (rad/s) available from drivetrain into axle "/1 -> Demux1/1
  Demux1/1 -> Add2/2
  Mux/1 -> drive torque (Nm) speed (rad/s) brake torque (Nm) req'd from drivetrain into axle/1
  Gain1/1 -> Add/2
  Add/1 -> Mux/1
  Add2/1 -> Gain2/1
  Gain2/1 -> Tire slip model/1(In1)
  Mux3/1 -> Scope/1, tractive force (N) brake force (N) linear speed achievable (m/s)/1
  Demux/2 -> axle input speed (rad/s)/1, Interia torque/1(车轮线速度 m/s), Interia torque1/1(车轮线速度 m/s)
  Interia torque/1(inertia torque (Nm)) -> Add2/1, Add/1
  Demux/3 -> Gain4/1
  Gain4/1 -> Add1/1
  Interia torque1/1(inertia torque (Nm)) -> Add3/1, Add1/2
  axle input speed (rad/s)/1 -> Switch1/2, Mux/2
  Switch1/1 -> Mux/3
  Constant/1 -> Switch1/3
  Add1/1 -> Switch1/1
  Saturation/1 -> Mux3/1
  Tire slip model/1(dri_force available in front wheel n) -> Saturation/1
  Tire slip model1/1(brk_force available in front wheel n) -> Saturation1/1
  Saturation1/1 -> Regenerative energy compute/1(motor brk force), Mux3/2
  Gain3/1 -> Tire slip model1/1(In1)
  Demux1/2 -> Add3/2
  Add3/1 -> Gain3/1
  Demux1/3 -> -/1
  -/1 -> Regenerative energy compute/3(spd2), Regenerative energy compute/2(spd), Mux3/3

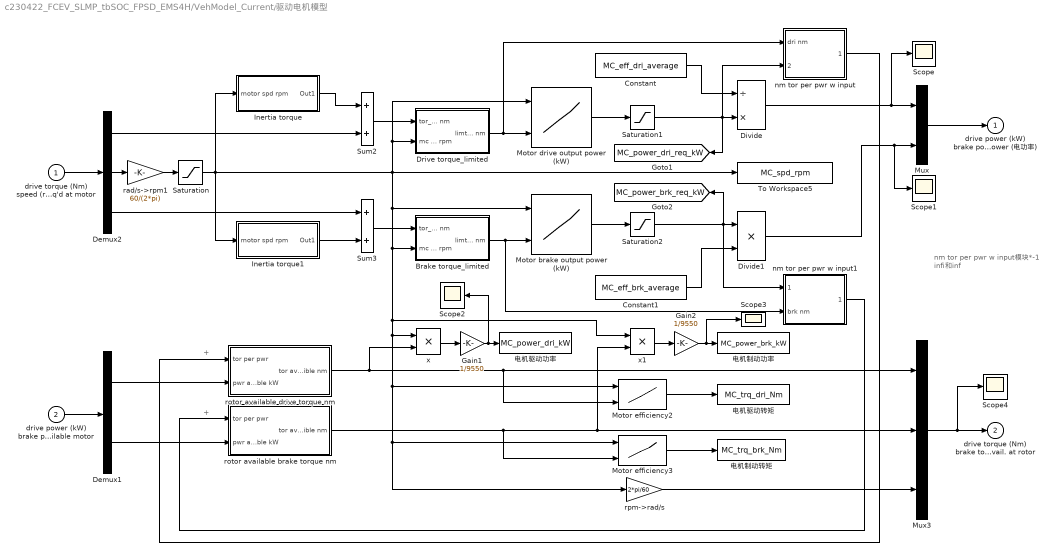
== system c230422_FCEV_SLMP_tbSOC_FPSD_EMS4H/VehModel_Current/驱动电机模型 ==
  note: +
  note: +
  note: nm tor per pwr w input模块*-1
      | infi和inf
  drive torque (Nm) speed (rad/s) brake torque (Nm) req'd at motor : Inport
  drive power (kW) brake power (kW) input available motor : Inport  Port=2
  Brake torque_limited : Subsystem
  Constant : Constant  Value=MC_eff_dri_average
  Constant1 : Constant  Value=MC_eff_brk_average
  Demux1 : Demux  Outputs=2
  Demux2 : Demux  Outputs=3
  Divide : Product  Inputs=/*
  Divide1 : Product  Inputs=**
  Drive torque_limited : Subsystem
  Gain1 : Gain  Gain=1/9550
  Gain2 : Gain  Gain=1/9550
  Inertia torque : Subsystem
  Inertia torque1 : Subsystem
  Motor brake output power (kW) : Lookup2D  RowIndex=MC_ori_spd_rpm*MC_spd_scale  ColumnIndex=MC_ori_trq_brk_Nm*MC_trq_scale  Table=MC_ori_power_brk_req_kW*MC_spd_scale*MC_trq_scale
  Motor drive output power (kW) : Lookup2D  RowIndex=MC_ori_spd_rpm*MC_spd_scale  ColumnIndex=MC_ori_trq_dri_Nm*MC_trq_scale  Table=MC_ori_power_dri_req_kW*MC_spd_scale*MC_trq_scale
  Motor efficiency2 : Lookup2D  RowIndex=MC_ori_spd_rpm*MC_spd_scale  ColumnIndex=MC_ori_trq_Nm*MC_trq_scale  Table=MC_ori_eff*MC_spd_scale*MC_trq_scale
  Motor efficiency3 : Lookup2D  RowIndex=MC_ori_spd_rpm*MC_spd_scale  ColumnIndex=MC_ori_trq_Nm*MC_trq_scale  Table=MC_ori_eff*MC_spd_scale*MC_trq_scale
  Mux : Mux  Inputs=2
  Mux3 : Mux  Inputs=3
  Saturation : Saturate  UpperLimit=MC_spd_max_rpm  LowerLimit=MC_spd_min_rpm
  Saturation1 : Saturate  UpperLimit=MC_power_max_kW  LowerLimit=0  LinearizeAsGain=off
  Saturation2 : Saturate  UpperLimit=0  LowerLimit=-MC_power_max_kW
  Scope{,1..4} (5 alike) : Scope
  Sum2 : Sum  InputSameDT=on  SaturateOnIntegerOverflow=on  OutDataTypeStr=Inherit: Same as first input
  Sum3 : Sum  InputSameDT=on  SaturateOnIntegerOverflow=on  OutDataTypeStr=Inherit: Same as first input
  To Workspace5 : ToWorkspace  VariableName=MC_spd_rpm  SampleTime=-1
  nm tor per pwr w input : Subsystem
  nm tor per pwr w input1 : Subsystem
  rad/s->rpm1 : Gain  Gain=60/(2*pi)
  rotor available brake torque nm : Subsystem
  rotor available drive torque nm : Subsystem
  rpm->rad/s : Gain  Gain=2*pi/60
  x : Product  Inputs=**
  x1 : Product  Inputs=**
  电机制动功率 : ToWorkspace  VariableName=MC_power_brk_kW  SampleTime=-1
  电机制动转矩 : ToWorkspace  VariableName=MC_trq_brk_Nm  SampleTime=-1
  电机驱动功率 : ToWorkspace  VariableName=MC_power_dri_kW  SampleTime=-1
  电机驱动转矩 : ToWorkspace  VariableName=MC_trq_dri_Nm  SampleTime=-1
  drive power (kW) brake power (kW) req'd motor input power (电功率) : Outport  InitialOutput=0
  drive torque (Nm) brake torque (Nm) speed avail (rad/s) avail. at rotor : Outport  Port=2  InitialOutput=0
  tag scope: MC_power_brk_req_kW=global, MC_power_dri_req_kW=global
  wires:
  drive torque (Nm) speed (rad/s) brake torque (Nm) req'd at motor/1 -> Demux2/1
  rad/s->rpm1/1 -> Saturation/1
  Demux2/2 -> rad/s->rpm1/1
  Demux2/1 -> Sum2/2
  Inertia torque/1(Out1) -> Sum2/1
  Sum2/1 -> Drive torque_limited/1(tor_req nm)
  Drive torque_limited/1(limted mc torque nm) -> Motor drive output power (kW)/2, nm tor per pwr w input/1(dri nm)
  Motor drive output power (kW)/1 -> Saturation1/1
  Constant/1 -> Divide/1
  Divide/1 -> Scope/1, Mux/1
  Mux/1 -> drive power (kW) brake power (kW) req'd motor input power (电功率)/1
  Demux2/3 -> Sum3/1
  Inertia torque1/1(Out1) -> Sum3/2
  Sum3/1 -> Brake torque_limited/1(tor_req nm)
  Motor brake output power (kW)/1 -> Saturation2/1
  Saturation2/1 -> [MC_power_brk_req_kW], nm tor per pwr w input1/1(pwr brk kW), Divide1/1
  Constant1/1 -> Divide1/2
  Divide1/1 -> Scope1/1, Mux/2
  drive power (kW) brake power (kW) input available motor/1 -> Demux1/1
  Saturation1/1 -> nm tor per pwr w input/2(pwr dri kW), [MC_power_dri_req_kW], Divide/2
  Demux1/1 -> rotor available drive torque nm/2(pwr available kW)
  nm tor per pwr w input/1(tor per pwr) -> rotor available drive torque nm/1(tor per pwr)
  Demux1/2 -> rotor available brake torque nm/2(pwr available kW)
  nm tor per pwr w input1/1(tor per pwr) -> rotor available brake torque nm/1(tor per pwr)
  rotor available brake torque nm/1(tor avaible nm) -> Motor efficiency3/2, x1/2, Mux3/2
  rotor available drive torque nm/1(tor avaible nm) -> Motor efficiency2/2, Mux3/1, x/2
  rpm->rad/s/1 -> Mux3/3
  Motor efficiency3/1 -> 电机制动转矩/1
  Motor efficiency2/1 -> 电机驱动转矩/1
  Brake torque_limited/1(limted mc torque nm) -> nm tor per pwr w input1/2(brk nm), Motor brake output power (kW)/2
  Gain1/1 -> Scope2/1, 电机驱动功率/1
  x/1 -> Gain1/1
  Gain2/1 -> Scope3/1, 电机制动功率/1
  x1/1 -> Gain2/1
  Saturation/1 -> Inertia torque1/1(motor spd rpm), x1/1, x/1, Motor efficiency2/1, Motor efficiency3/1, rpm->rad/s/1, Brake torque_limited/2(mc spd rpm), Motor brake output power (kW)/1, To Workspace5/1, Motor drive output power (kW)/1, Drive torque_limited/2(mc spd rpm), Inertia torque/1(motor spd rpm)
  Mux3/1 -> Scope4/1, drive torque (Nm) brake torque (Nm) speed avail (rad/s) avail. at rotor/1

== system c230422_FCEV_SLMP_tbSOC_FPSD_EMS4H/Subsystem3/FcDegCountingSubSys/Subsystem ==
  Enable : EnablePort
  Add : Sum
  Constant : Constant
  Memory : Memory
  u : Outport
  wires:
  Constant/1 -> Add/1
  Add/1 -> Memory/1
  Memory/1 -> Add/2, u/1

== system c230422_FCEV_SLMP_tbSOC_FPSD_EMS4H/Subsystem3/FcDegCountingSubSys/Subsystem1 ==
  Enable : EnablePort
  Add : Sum
  Constant : Constant
  Memory : Memory
  u : Outport
  wires:
  Memory/1 -> u/1, Add/2
  Add/1 -> Memory/1
  Constant/1 -> Add/1

== system c230422_FCEV_SLMP_tbSOC_FPSD_EMS4H/Subsystem4/VehModel_Pred+1/Power bus ==
  note: -
  note: +
  note: 需求制动功率
  note: 需求驱动功率
  drive power (kW) brake power (kW) req at power bus : Inport
  Constant1 : Constant  Value=DCAC_eff
  Demux2 : Demux  Outputs=2
  Divide : Product  Inputs=*/
  Divide1 : Product  Inputs=**
  Saturation : Saturate  UpperLimit=0  LowerLimit=-inf
  Saturation1 : Saturate  UpperLimit=inf  LowerLimit=0
  Switch1 : Switch  Criteria=u2 > Threshold  SaturateOnIntegerOverflow=off  InputSameDT=off
  drive power (kW)/brake power (kW) req from power sources : Outport
  wires:
  Constant1/1 -> Divide1/2, Divide/2
  Divide/1 -> Saturation1/1
  Divide1/1 -> Saturation/1
  drive power (kW) brake power (kW) req at power bus/1 -> Demux2/1
  Demux2/2 -> Divide1/1
  Saturation1/1 -> Switch1/2, Switch1/1
  Switch1/1 -> drive power (kW)/brake power (kW) req from power sources/1
  Saturation/1 -> Switch1/3
  Demux2/1 -> Divide/1

== system c230422_FCEV_SLMP_tbSOC_FPSD_EMS4H/Subsystem4/VehModel_Pred+1/主减及变速器模型 ==
  drive torque (Nm) speed (rad/s) brake torque (Nm) req'd at output side of final drive : Inport
  " Effect of inertia (Nm)1" : Subsystem
  Demux4 : Demux  Outputs=3
  Effect of inertia (Nm) : Subsystem
  Gain1 : Gain  Gain=1/Veh_final_drive_ratio
  Gain2 : Gain  Gain=1/Veh_final_drive_ratio
  Gain3 : Gain  Gain=Veh_final_drive_ratio  SaturateOnIntegerOverflow=on  OutDataTypeStr=Inherit: Same as input  ParamDataTypeStr=Inherit: Same as input
  Mux4 : Mux  Inputs=3
  Sum : Sum  Inputs=+++  InputSameDT=on  SaturateOnIntegerOverflow=on  OutDataTypeStr=Inherit: Same as first input
  Sum3 : Sum  Inputs=+++  InputSameDT=on  SaturateOnIntegerOverflow=on  OutDataTypeStr=Inherit: Same as first input
  loss (Nm) : Subsystem
  loss (Nm)1 : Subsystem
  drive torque (Nm) speed (rad/s) brike torque (Nm) req'd at input side of final drive : Outport  InitialOutput=0
  wires:
  Demux4/2 -> Effect of inertia (Nm)/1(fd input speed (rad/s)), " Effect of inertia (Nm)1"/1(In1), Gain3/1
  Demux4/1 -> loss (Nm)/1("drive torque (Nm) "), Gain1/1
  Mux4/1 -> drive torque (Nm) speed (rad/s) brike torque (Nm) req'd at input side of final drive/1
  drive torque (Nm) speed (rad/s) brake torque (Nm) req'd at output side of final drive/1 -> Demux4/1
  Effect of inertia (Nm)/1(drag torque (Nm)) -> Sum/2
  loss (Nm)/1(drag torque (Nm)) -> Sum/1
  Gain1/1 -> Sum/3
  Sum/1 -> Mux4/1
  Gain3/1 -> Mux4/2
  " Effect of inertia (Nm)1"/1(Out1) -> Sum3/2
  loss (Nm)1/1(drag torque (Nm)) -> Sum3/3
  Demux4/3 -> Gain2/1, loss (Nm)1/1("drive torque (Nm) ")
  Gain2/1 -> Sum3/1
  Sum3/1 -> Mux4/3

== system c230422_FCEV_SLMP_tbSOC_FPSD_EMS4H/Subsystem4/VehModel_Pred+1/整车动力学模型 ==
  需求车速 km/h : Inport
  Add1 : Sum  Inputs=++++
  Mux : Mux  Inputs=3
  compute of front axle brk from motor : Subsystem
  kmph->m/s : Gain  Gain=1/3.6
  加速阻力 : Subsystem
  坡度 : Constant  Value=0
  坡道阻力 : Subsystem
  平均车速 km/h : Scope
  整车需求驱动力 : Scope
  滚动阻力 : Subsystem
  空气阻力 : Subsystem
  需求驱动力N 目标车速m/s 需求制动力N : Outport
  wires:
  滚动阻力/1(滚动阻力 N) -> Add1/1
  坡道阻力/1(坡道阻力 N) -> Add1/2
  空气阻力/1(空气阻力 N) -> Add1/3
  加速阻力/1(加速阻力 N) -> Add1/4
  Add1/1 -> 整车需求驱动力/1, Mux/1
  Mux/1 -> 需求驱动力N 目标车速m/s 需求制动力N/1
  坡度/1 -> 坡道阻力/2(预测坡度), 滚动阻力/2(预测坡度)
  kmph->m/s/1 -> Mux/2
  需求车速 km/h/1 -> compute of front axle brk from motor/1(平均车速 km/h), kmph->m/s/1, 平均车速 km/h/1, 加速阻力/1(车速 km/h), 空气阻力/1(veh_spd km/h), 滚动阻力/1(车辆平均车速 km/h), 坡道阻力/1(车辆平均车速1)
  compute of front axle brk from motor/1(veh_front_axle_motor_brk) -> Mux/3

== system c230422_FCEV_SLMP_tbSOC_FPSD_EMS4H/Subsystem4/VehModel_Pred+1/车轮模型 ==
  "tractive force, brake force and speed req'd of tire/road interface 需求驱动力N 目标车速m/s 需求制动力N" : Inport
  Add : Sum
  Add1 : Sum
  Constant : Constant  Value=0
  Demux : Demux  Outputs=3
  Gain1 : Gain  Gain=Veh_wheel_radius_m
  Gain4 : Gain  Gain=Veh_wheel_radius_m
  Interia torque : Subsystem
  Interia torque1 : Subsystem
  Mux : Mux  Inputs=3
  Switch1 : Switch  Criteria=u2 > Threshold  Threshold=15  SaturateOnIntegerOverflow=off  InputSameDT=off
  axle input speed (rad/s) : Gain  Gain=1/Veh_wheel_radius_m
  drive torque (Nm) speed (rad/s) brake torque (Nm) req'd from drivetrain into axle : Outport  InitialOutput=0
  wires:
  Demux/1 -> Gain1/1
  "tractive force, brake force and speed req'd of tire/road interface 需求驱动力N 目标车速m/s 需求制动力N"/1 -> Demux/1
  Mux/1 -> drive torque (Nm) speed (rad/s) brake torque (Nm) req'd from drivetrain into axle/1
  Gain1/1 -> Add/2
  Add/1 -> Mux/1
  Demux/2 -> axle input speed (rad/s)/1, Interia torque/1(车轮线速度 m/s), Interia torque1/1(车轮线速度 m/s)
  Interia torque/1(inertia torque (Nm)) -> Add/1
  Demux/3 -> Gain4/1
  Gain4/1 -> Add1/1
  Interia torque1/1(inertia torque (Nm)) -> Add1/2
  axle input speed (rad/s)/1 -> Switch1/2, Mux/2
  Switch1/1 -> Mux/3
  Constant/1 -> Switch1/3
  Add1/1 -> Switch1/1

== system c230422_FCEV_SLMP_tbSOC_FPSD_EMS4H/Subsystem4/VehModel_Pred+1/驱动电机模型 ==
  note: nm tor per pwr w input模块*-1
      | infi和inf
  drive torque (Nm) speed (rad/s) brake torque (Nm) req'd at motor : Inport
  Brake torque_limited : Subsystem
  Constant : Constant  Value=MC_eff_dri_average
  Constant1 : Constant  Value=MC_eff_brk_average
  Demux2 : Demux  Outputs=3
  Divide : Product  Inputs=/*
  Divide1 : Product  Inputs=**
  Drive torque_limited : Subsystem
  Inertia torque : Subsystem
  Inertia torque1 : Subsystem
  Motor brake output power (kW) : Lookup2D  RowIndex=MC_ori_spd_rpm*MC_spd_scale  ColumnIndex=MC_ori_trq_brk_Nm*MC_trq_scale  Table=MC_ori_power_brk_req_kW*MC_spd_scale*MC_trq_scale
  Motor drive output power (kW) : Lookup2D  RowIndex=MC_ori_spd_rpm*MC_spd_scale  ColumnIndex=MC_ori_trq_dri_Nm*MC_trq_scale  Table=MC_ori_power_dri_req_kW*MC_spd_scale*MC_trq_scale
  Mux : Mux  Inputs=2
  Saturation : Saturate  UpperLimit=MC_spd_max_rpm  LowerLimit=MC_spd_min_rpm
  Saturation1 : Saturate  UpperLimit=MC_power_max_kW  LowerLimit=0  LinearizeAsGain=off
  Saturation2 : Saturate  UpperLimit=0  LowerLimit=-MC_power_max_kW
  Sum2 : Sum  InputSameDT=on  SaturateOnIntegerOverflow=on  OutDataTypeStr=Inherit: Same as first input
  Sum3 : Sum  InputSameDT=on  SaturateOnIntegerOverflow=on  OutDataTypeStr=Inherit: Same as first input
  rad/s->rpm1 : Gain  Gain=60/(2*pi)
  drive power (kW) brake power (kW) req'd motor input power (电功率) : Outport  InitialOutput=0
  wires:
  drive torque (Nm) speed (rad/s) brake torque (Nm) req'd at motor/1 -> Demux2/1
  rad/s->rpm1/1 -> Saturation/1
  Demux2/2 -> rad/s->rpm1/1
  Demux2/1 -> Sum2/2
  Inertia torque/1(Out1) -> Sum2/1
  Sum2/1 -> Drive torque_limited/1(tor_req nm)
  Drive torque_limited/1(limted mc torque nm) -> Motor drive output power (kW)/2
  Motor drive output power (kW)/1 -> Saturation1/1
  Constant/1 -> Divide/1
  Divide/1 -> Mux/1
  Mux/1 -> drive power (kW) brake power (kW) req'd motor input power (电功率)/1
  Demux2/3 -> Sum3/1
  Inertia torque1/1(Out1) -> Sum3/2
  Sum3/1 -> Brake torque_limited/1(tor_req nm)
  Motor brake output power (kW)/1 -> Saturation2/1
  Saturation2/1 -> Divide1/1
  Constant1/1 -> Divide1/2
  Divide1/1 -> Mux/2
  Saturation1/1 -> Divide/2
  Brake torque_limited/1(limted mc torque nm) -> Motor brake output power (kW)/2
  Saturation/1 -> Inertia torque1/1(motor spd rpm), Brake torque_limited/2(mc spd rpm), Motor brake output power (kW)/1, Motor drive output power (kW)/1, Drive torque_limited/2(mc spd rpm), Inertia torque/1(motor spd rpm)

== system c230422_FCEV_SLMP_tbSOC_FPSD_EMS4H/Subsystem4/VehModel_Pred+2/Power bus ==
  note: -
  note: +
  note: 需求制动功率
  note: 需求驱动功率
  drive power (kW) brake power (kW) req at power bus : Inport
  Constant1 : Constant  Value=DCAC_eff
  Demux2 : Demux  Outputs=2
  Divide : Product  Inputs=*/
  Divide1 : Product  Inputs=**
  Saturation : Saturate  UpperLimit=0  LowerLimit=-inf
  Saturation1 : Saturate  UpperLimit=inf  LowerLimit=0
  Switch1 : Switch  Criteria=u2 > Threshold  SaturateOnIntegerOverflow=off  InputSameDT=off
  drive power (kW)/brake power (kW) req from power sources : Outport
  wires:
  Constant1/1 -> Divide1/2, Divide/2
  Divide/1 -> Saturation1/1
  Divide1/1 -> Saturation/1
  drive power (kW) brake power (kW) req at power bus/1 -> Demux2/1
  Demux2/2 -> Divide1/1
  Saturation1/1 -> Switch1/2, Switch1/1
  Switch1/1 -> drive power (kW)/brake power (kW) req from power sources/1
  Saturation/1 -> Switch1/3
  Demux2/1 -> Divide/1
